simulink model "FAST_EMPC"  (R2021a)
settings: Solver=ode4  StartTime=0.0  StopTime=TMax  FixedStep=DT  MaxStep=DT  RelTol=1e-3  EnableMultiTasking=on
values from neighbouring files (symbols this model uses):
  Drivetrain =     [NREL5MW.mat]
  luenGainDisc = place(sys_tower_fa_d_obsv.A',sys_tower_fa_d_obsv.C',luenPolesDisc)'    [Init_FAST_EMPC.m]
  Parameters =     [Parameters.mat]
  RPM_Init = 9.4965    [Init_FAST_EMPC.m]
  sys_tower_fa_d_obsv = c2d(sys_tower_ss_obsv,Parameters.TsObsv,'tustin')    [Init_FAST_EMPC.m]
  sys_tower_fa_d_obsv_mode = c2d(sys_tower_ss_obsv_mode,Parameters.TsObsv,'tustin')    [Init_FAST_EMPC.m]
undefined symbols (not defined in the file or in its folder): EMPCController_Tower, luenGainDisc2, luenGainDisc_comp, OutList, strmatch, sys_tower_fa_d_obsv2, sys_tower_fa_d_obsv_comp
libraries: dspstat3 x8
(part 1 of 2)
settings Model: PauseTimes=360  Creator=bjonkman  LastModifiedBy=zfeng1
settings SolverCC: AlgebraicLoopSolver=TrustRegion
settings DataIOCC: LimitDataPoints=on  SaveFormat=Array  SignalLoggingSaveFormat=ModelDataLogs  SaveOutput=off  SaveTime=off  ReturnWorkspaceOutputs=off  SignalLoggingName=sigsOut  LoggingToFile=on  LoggingFileName=FAST_EMPC_log/220905/[220905][171055]sim_log.mat
settings OptimizationCC: ExpressionDepthLimit=2147483647  LifeSpan=inf
settings DebuggingCC: SaveWithParameterizedLinksMsg=none  UnderspecifiedInitializationDetection=Classic  MergeDetectMultiDrivingBlocksExec=none  SignalResolutionControl=TryResolveAllWithWarning  MultiTaskDSMMsg=warning  MultiTaskCondExecSysMsg=none  MultiTaskRateTransMsg=warning  FcnCallInpInsideContextMsg=warning  StateNameClashWarn=warning  SFUnexpectedBacktrackingDiag=warning  SFNoUnconditionalDefaultTransitionDiag=warning  SFExecutionAtInitializationDiag=none  SFMachineParentedDataDiag=warning  ArithmeticOperatorsInVariantConditions=warning
settings HardwareCC: ProdBitPerPointer=32  ProdBitPerSizeT=32  ProdBitPerPtrDiffT=32  ProdLargestAtomicFloat=None  ProdIntDivRoundTo=Undefined  ProdEndianess=Unspecified  ProdWordSize=32  ProdHWDeviceType=32-bit Generic  TargetUnknown=on
settings ModelReferenceCC: PropagateSignalLabelsOutOfModel=off
settings SFSimCC: SimUseLocalCustomCode=off  CustomCodeUndefinedFunction=UseInterfaceOnly
settings RTWCC: RTWUseLocalCustomCode=off
settings CodeAppCC: StateflowObjectComments=on
settings GRTTargetCC: TargetLangStandard=C89/C90 (ANSI)  CombineOutputUpdateFcns=off  GRTInterface=on
settings ConfigComp: CovMetricSettings=dw  CovSaveCumulativeToWorkspaceVar=on  CovSaveSingleToWorkspaceVar=on  CovExternalEMLEnable=off

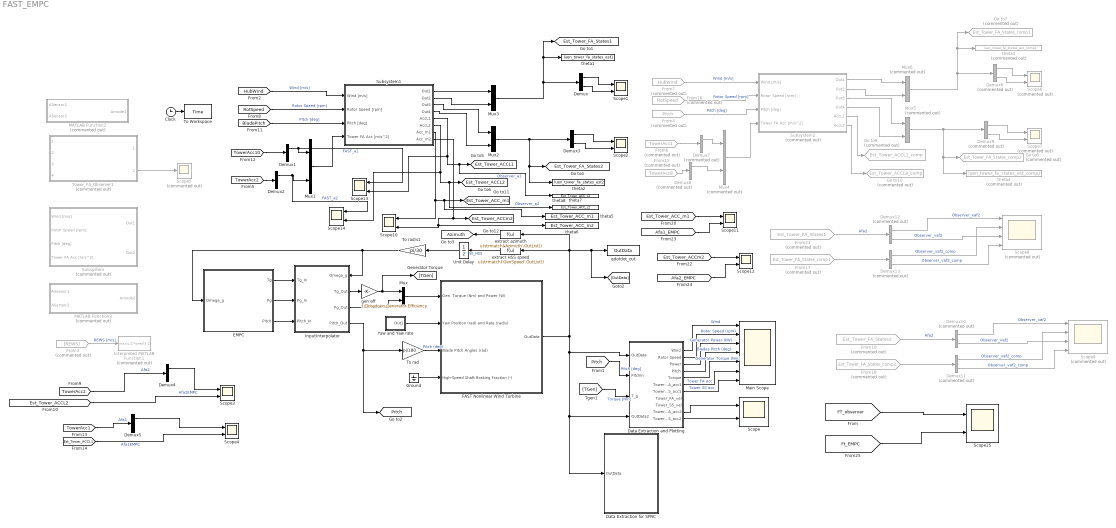
== system FAST_EMPC ==
  Clock : Clock
  Data Extraction and Plotting : Subsystem
  Data Extraction for SPRC : Subsystem
  Demux{,1..5} (6 alike) : Demux  Outputs=2
  Demux{6..13} (8 alike) : Demux  Commented=on  Outputs=2
  EMPC : Subsystem
  FAST Nonlinear Wind Turbine : Subsystem  mask(FAST Nonlinear Wind Turbine){}
      mask help: This block contains the FAST S-Function.
      mask init:
      | clear FAST_SFunc
  From15 : From  Commented=on  GotoTag=TowerAcc8  TagVisibility=global
  From16 : From  Commented=on  GotoTag=RotSpeed  TagVisibility=global
  From17 : From  Commented=on  GotoTag=Est_Tower_FA_States_comp1  TagVisibility=global
  From18 : From  Commented=on  GotoTag=Est_Tower_FA_States_comp2  TagVisibility=global
  From19 : From  Commented=on  GotoTag=Est_Tower_FA_States2  TagVisibility=global
  From21 : From  Commented=on  GotoTag=Est_Tower_FA_States1  TagVisibility=global
  From3 : From  Commented=on  GotoTag=REWS  TagVisibility=global
  From4 : From  Commented=on  GotoTag=Pitch  TagVisibility=global
  From6 : From  Commented=on  GotoTag=TowerAcc1  TagVisibility=global
  From7 : From  Commented=on  GotoTag=HubWind  TagVisibility=global
  Go to10 : Goto  Commented=on  GotoTag=Est_Tower_ACCL8_comp  TagVisibility=global
  Go to7 : Goto  Commented=on  GotoTag=Est_Tower_FA_States_comp1  TagVisibility=global
  Go to8 : Goto  Commented=on  GotoTag=Est_Tower_FA_States_comp2  TagVisibility=global
  Go to9 : Goto  Commented=on  GotoTag=Est_Tower_ACCL1_comp  TagVisibility=global
  Ground : Ground
  InputInterpolator : Subsystem
      settings: PortSchema="{\"entries\":[{\"content\":{\"sides\":[{\"content\":{\"connectorIds\":[\"In1\",\"In2\",\"In3\"]},\"type\":\"ConnectorPlacement.EquallySpacedRectSide\",\"uuid\":\"eea9236e-1f3f-4277-abdd-d5dd724ebb06\"},{\"content\":{\"connectorIds\":[\"In4\",\"Out1\",\"Out2\",\"Out3\"],\"side\":\"RIGHT\"},\"type\":\"ConnectorPlacement.EquallySpacedRectSide\",\"uuid\":\"af4b7fb0-ea5a-4e1a-9e28-eb831b9d8a57\"},{\"content\":{\"connectorIds\":[],\"side\":\"TOP\"},\"type\":\"ConnectorPlacement.EquallySpacedRectSide\",\"uuid\":\"835f85ff-c21c-4848-971b-3562e8e2ecd8\"},{\"content\":{\"connectorIds\":[],\"side\":\"BOTTOM\"},\"type\":\"ConnectorPlacement.EquallySpacedRectSide\",\"uuid\":\"cf59863e-7ec1-458a-af15-cb3c9fb145f1\"}]},\"type\":\"ConnectorPlacement.EquallySpacedConnector\",\"uuid\":\"4273e109-3171-481c-9f40-fed22461b3da\"}],\"packageUris\":[\"http://schema.mathworks.com/mf0/Connector/R2020b\"],\"version\":\"1.0\"}"
  Interpreted MATLAB Function1 : MATLABFcn  Commented=on  MATLABFcn=max(u,4)*ones(3,1)  OutputDimensions=3
  MATLAB Function2 : MATLAB Function  Commented=on  TreatAsAtomicUnit=on
  MATLAB Function3 : MATLAB Function  Commented=on  TreatAsAtomicUnit=on
  Main Scope : Scope  NumInputPorts=7
      settings: Tag=Scope
  Mux{,1..3} (4 alike) : Mux  Inputs=2
  Mux4 : Mux  Commented=on  Inputs=2
  Mux5 : Mux  Commented=on  Inputs=2
  Mux6 : Mux  Commented=on  Inputs=2
  Scope{,1..4,10..15} (11 alike) : Scope  NumInputPorts=2
  Scope5 : Scope  Commented=on
  Scope6 : Scope  Commented=on  NumInputPorts=2
  Scope7 : Scope  Commented=on  NumInputPorts=2
  Scope8 : Scope  Commented=on  NumInputPorts=4
  Scope9 : Scope  Commented=on  NumInputPorts=4
  Subsystem : Subsystem  Commented=on
  Subsystem1 : Subsystem
  Subsystem2 : Subsystem  Commented=on
  To Workspace : ToWorkspace  VariableName=Time  SampleTime=-1
  To rad : Gain  Gain=pi/180
  To rad/s1 : Gain  Gain=pi/30
  Tower_FA_Observer1 : Subsystem  Commented=on  ReferencedSubsystem=Luenberger_Tower_FA_Observer
  Unit Delay : UnitDelay  InitialCondition=RPM_Init*Drivetrain.Gearbox.Ratio  SampleTime=-1  HasFrameUpgradeWarning=on
  Yaw and Yaw rate : Subsystem
  extract HSS speed : Fcn  Expr=u(strmatch('GenSpeed',OutList))
  extract azimuth : Fcn  Expr=u(strmatch('Azimuth',OutList))
  gen eff : Gain  Gain=1/Drivetrain.Generator.Efficiency
  qdotdot_out : ToWorkspace  VariableName=OutData  SampleTime=-1
  theta1 : ToWorkspace  VariableName=luen_tower_fa_states_est1  SaveFormat=Structure With Time  SampleTime=-1
      settings: MaxDataPoints=Inf  Decimation=3
  theta2 : ToWorkspace  VariableName=luen_tower_fa_states_est2  SaveFormat=Structure With Time  SampleTime=-1
      settings: MaxDataPoints=Inf  Decimation=3
  theta3 : ToWorkspace  Commented=on  VariableName=luen_tower_fa_states_est_comp1  SaveFormat=Structure With Time  SampleTime=-1
      settings: MaxDataPoints=Inf  Decimation=3
  theta4 : ToWorkspace  Commented=on  VariableName=luen_tower_fa_states_est_comp2  SaveFormat=Structure With Time  SampleTime=-1
      settings: MaxDataPoints=Inf  Decimation=3
  theta5 : ToWorkspace  VariableName=Est_Tower_ACC_m1  SaveFormat=Structure With Time  SampleTime=-1
      settings: MaxDataPoints=Inf  Decimation=3
  theta6 : ToWorkspace  VariableName=Est_Tower_ACC_m2  SaveFormat=Structure With Time  SampleTime=-1
      settings: MaxDataPoints=Inf  Decimation=3
  theta7 : ToWorkspace  VariableName=Est_Tower_ACC_L1  SaveFormat=Structure With Time  SampleTime=-1
      settings: MaxDataPoints=Inf  Decimation=3
  theta8 : ToWorkspace  VariableName=Est_Tower_ACC_L2  SaveFormat=Structure With Time  SampleTime=-1
      settings: MaxDataPoints=Inf  Decimation=3
  tag scope: Azimuth=global, Est_Tower_ACCL1=global, Est_Tower_ACCL2=global, Est_Tower_ACC_m1=global, Est_Tower_ACCm2=global, Est_Tower_FA_States1=global, Est_Tower_FA_States2=global, Pitch=global
  wires:
  Clock/1 -> To Workspace/1
  Ground/1 -> FAST Nonlinear Wind Turbine/4(High-Speed Shaft Braking Fraction (-))
  Yaw and Yaw rate/1(Out1) -> FAST Nonlinear Wind Turbine/2(Yaw Position (rad) and Rate (rad/s))
  Mux/1 -> FAST Nonlinear Wind Turbine/1(Gen. Torque (Nm) and Power (W))
  Data Extraction and Plotting/7(Tower_SS_acc1) -> Main Scope/7  "Tower SS acc"
  Data Extraction and Plotting/2(Rotor Speed) -> Main Scope/2  "Rotor Speed (rpm)"
  Data Extraction and Plotting/3(Power) -> Main Scope/3  "Generator Power (kW)"
  Data Extraction and Plotting/4(Pitch) -> Main Scope/4  "Blades Pitch (deg)"
  Data Extraction and Plotting/5(Torque) -> Main Scope/5  "Generator Torque (Nm)"
  Data Extraction and Plotting/6(Tower_FA_acc1) -> Main Scope/6  "Tower FA acc"
  [TGen] -> Data Extraction and Plotting/3(T_g)  "Torque [Nm]"
  Data Extraction and Plotting/1(Wind) -> Main Scope/1  "Wind"
  [Pitch] -> Data Extraction and Plotting/2(PitchIn)  "Pitch [deg]"
  Unit Delay/1 -> To rad/s1/1
  extract azimuth/1 -> [Azimuth]
  extract HSS speed/1 -> Unit Delay/1  "W_HSS"
  To rad/s1/1 -> EMPC/1(Omega_g), InputInterpolator/4(Omega_g)
  InputInterpolator/1(Tg_Out) -> gen eff/1
  gen eff/1 -> Mux/1, [TGen]
  InputInterpolator/2(Pg_Out) -> Mux/2
  To rad/1 -> FAST Nonlinear Wind Turbine/3(Blade Pitch Angles (rad))  "Pitch (deg)"
  InputInterpolator/3(Pitch_Out) -> [Pitch], To rad/1
  EMPC/1(Tg) -> InputInterpolator/1(Tg_In)
  EMPC/2(Pg) -> InputInterpolator/2(Pg_In)
  EMPC/3(Pitch) -> InputInterpolator/3(Pitch_In)
  [RotSpeed] -> Subsystem1/2(Rotor Speed [rpm])  "Rotor Speed [rpm]"
  [HubWind] -> Subsystem1/1(Wind [m/s])  "Wind [m/s]"
  Subsystem1/1(Out1) -> Mux3/1
  Subsystem1/2(Out2) -> Mux3/2
  Mux3/1 -> Demux/1, [Est_Tower_FA_States1], theta1/1
  From3/1 -> Interpreted MATLAB Function1/1  "REWS [m/s]"
  FAST Nonlinear Wind Turbine/1(OutData) -> Data Extraction for SPRC/1(OutData), Data Extraction and Plotting/4(OutData2), Data Extraction and Plotting/1(OutData), extract azimuth/1, extract HSS speed/1, [OutData], qdotdot_out/1
  Data Extraction and Plotting/10(Tower_FA_acc2) -> Scope/1
  Data Extraction and Plotting/11(Tower_SS_acc2) -> Scope/2
  Demux3/1 -> Scope2/1
  Demux3/2 -> Scope2/2
  Demux/1 -> Scope1/1
  Demux/2 -> Scope1/2
  [TowerAcc2] -> Demux4/1  "Afa2"
  [Est_Tower_ACCL2] -> Scope3/2  "Afa2EMPC"
  [TowerAcc1] -> Demux5/1  "Afa1"
  [Est_Tower_ACCL1] -> Scope4/2  "Afa1EMPC"
  Tower_FA_Observer1/2 -> Scope5/1
  [BladePitch] -> Subsystem1/3(Pitch [deg])  "Pitch [deg]"
  Mux1/1 -> Subsystem1/4(Tower FA Acc [m/s^2])
  [TowerAcc10] -> Demux1/1
  [TowerAcc2] -> Demux2/1
  Subsystem1/4(Out4) -> Mux2/2
  Subsystem1/3(Out3) -> Mux2/1
  Mux2/1 -> theta2/1, [Est_Tower_FA_States2], Demux3/1
  Demux2/1 -> Scope14/1, Mux1/2  "FAST_a2"
  Demux1/1 -> Scope13/1, Mux1/1  "FAST_a1"
  Subsystem1/5(AccL1) -> Scope13/2, theta7/1, [Est_Tower_ACCL1]  "Observer_a1"
  Subsystem1/6(AccL2) -> Scope14/2, theta8/1, [Est_Tower_ACCL2]  "Observer_a2"
  Demux4/1 -> Scope3/1
  Demux5/1 -> Scope4/1
  Subsystem2/6(AccL2) -> Go to10/1
  Subsystem2/5(AccL1) -> Go to9/1
  Demux8/1 -> Mux4/2
  From6/1 -> Demux7/1
  Subsystem2/4(Out4) -> Mux5/2
  From15/1 -> Demux8/1
  Subsystem2/3(Out3) -> Mux5/1
  Mux4/1 -> Subsystem2/4(Tower FA Acc [m/s^2])
  Mux5/1 -> theta4/1, Go to8/1, Demux9/1
  Subsystem2/2(Out2) -> Mux6/2
  Subsystem2/1(Out1) -> Mux6/1
  Demux7/1 -> Mux4/1
  From4/1 -> Subsystem2/3(Pitch [deg])  "Pitch [deg]"
  From16/1 -> Subsystem2/2(Rotor Speed [rpm])  "Rotor Speed [rpm]"
  From7/1 -> Subsystem2/1(Wind [m/s])  "Wind [m/s]"
  Demux9/1 -> Scope7/1
  Demux6/1 -> Scope6/1
  Mux6/1 -> Demux6/1, Go to7/1, theta3/1
  Demux6/2 -> Scope6/2
  Demux9/2 -> Scope7/2
  From17/1 -> Demux13/1
  From21/1 -> Demux12/1  "Afa2"
  Demux12/1 -> Scope8/1  "Observer_xaf2"
  Demux13/1 -> Scope8/2  "Observer_xaf2_comp"
  Demux12/2 -> Scope8/3  "Observer_vaf2"
  Demux13/2 -> Scope8/4  "Observer_vaf2_comp"
  Demux11/2 -> Scope9/4  "Observer_vaf2_comp"
  Demux10/1 -> Scope9/1  "Observer_xaf2"
  From19/1 -> Demux10/1  "Afa2"
  Demux11/1 -> Scope9/2  "Observer_xaf2_comp"
  From18/1 -> Demux11/1
  Demux10/2 -> Scope9/3  "Observer_vaf2"
  Subsystem1/7(Acc_m1) -> theta5/1, [Est_Tower_ACC_m1], Scope10/1
  [Est_Tower_ACC_m1] -> Scope11/1
  [Est_Tower_ACCm2] -> Scope12/1
  [Afa1_EMPC] -> Scope11/2
  [Afa2_EMPC] -> Scope12/2
  Subsystem1/8(Acc_m2) -> [Est_Tower_ACCm2], Scope10/2, theta6/1
  [FT_observer] -> Scope15/1
  [Ft_EMPC] -> Scope15/2

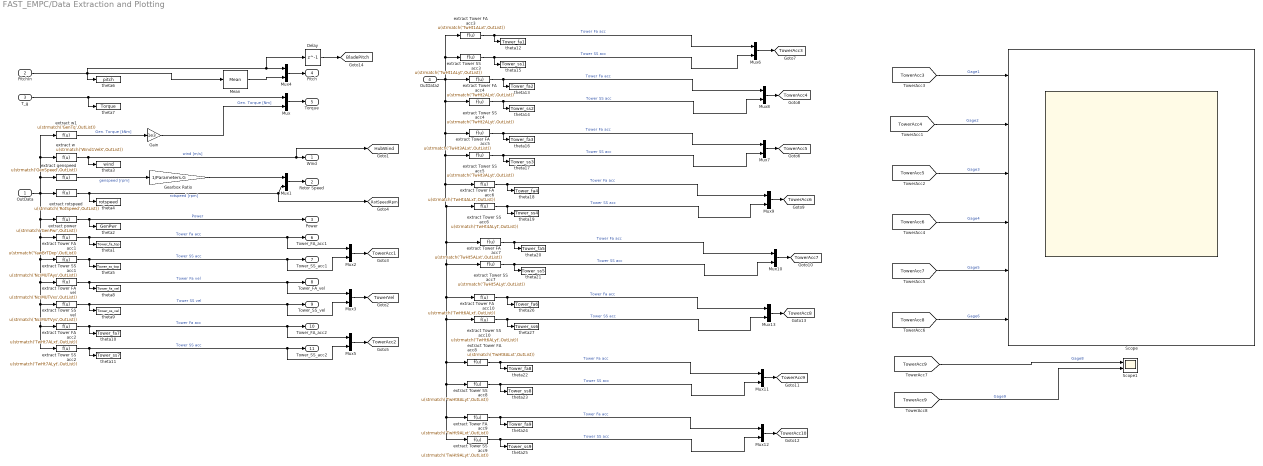
== system FAST_EMPC/Data Extraction and Plotting ==
  OutData : Inport
  PitchIn : Inport  Port=2
  T_g : Inport  Port=3
  OutData2 : Inport  Port=4
  Delay : Delay  DelayLength=1  InitialCondition=0
  Gain : Gain  Gain=1e3
  Gearbox Ratio : Gain  Gain=1/Parameters.G
  Mean : dspstat3/Mean  run=off  InputProcessing=Columns as channels (frame based)  reset_popup=None  directionMode=Each column  dimension=1  roiEnable=off  roiType=Rectangles  roiPortion=Entire ROI  roiOutput=Individual statistics for each ROI  roiFlag=off  roundingMode=Floor  overflowMode=off  outputDataTypeStr=Inherit: Same as accumulator  outputMin=[]  outputMax=[]  outputLastDataTypeStr=Inherit: Same as accumulator
  Mux{,1..13} (14 alike) : Mux  Inputs=2
  Scope : Scope  NumInputPorts=6
  Scope1 : Scope  NumInputPorts=2
  extract Tower FA acc1 : Fcn  Expr=u(strmatch('YawBrTDxp',OutList))
  extract Tower FA acc10 : Fcn  Expr=u(strmatch('TwHt6ALxt',OutList))
  extract Tower FA acc2 : Fcn  Expr=u(strmatch('TwHt7ALxt',OutList))
  extract Tower FA acc3 : Fcn  Expr=u(strmatch('TwHt1ALxt',OutList))
  extract Tower FA acc4 : Fcn  Expr=u(strmatch('TwHt2ALxt',OutList))
  extract Tower FA acc5 : Fcn  Expr=u(strmatch('TwHt3ALxt',OutList))
  extract Tower FA acc6 : Fcn  Expr=u(strmatch('TwHt4ALxt',OutList))
  extract Tower FA acc7 : Fcn  Expr=u(strmatch('TwHt5ALxt',OutList))
  extract Tower FA acc8 : Fcn  Expr=u(strmatch('TwHt8ALxt',OutList))
  extract Tower FA acc9 : Fcn  Expr=u(strmatch('TwHt9ALxt',OutList))
  extract Tower FA vel : Fcn  Expr=u(strmatch('NcIMUTVxs',OutList))
  extract Tower SS acc1 : Fcn  Expr=u(strmatch('NcIMUTAys',OutList))
  extract Tower SS acc10 : Fcn  Expr=u(strmatch('TwHt6ALyt',OutList))
  extract Tower SS acc2 : Fcn  Expr=u(strmatch('TwHt7ALyt',OutList))
  extract Tower SS acc3 : Fcn  Expr=u(strmatch('TwHt1ALyt',OutList))
  extract Tower SS acc4 : Fcn  Expr=u(strmatch('TwHt2ALyt',OutList))
  extract Tower SS acc5 : Fcn  Expr=u(strmatch('TwHt3ALyt',OutList))
  extract Tower SS acc6 : Fcn  Expr=u(strmatch('TwHt4ALyt',OutList))
  extract Tower SS acc7 : Fcn  Expr=u(strmatch('TwHt5ALyt',OutList))
  extract Tower SS acc8 : Fcn  Expr=u(strmatch('TwHt8ALyt',OutList))
  extract Tower SS acc9 : Fcn  Expr=u(strmatch('TwHt9ALyt',OutList))
  extract Tower SS vel : Fcn  Expr=u(strmatch('NcIMUTVys',OutList))
  extract genspeed : Fcn  Expr=u(strmatch('GenSpeed',OutList))
  extract power : Fcn  Expr=u(strmatch('GenPwr',OutList))
  extract rotspeed : Fcn  Expr=u(strmatch('RotSpeed',OutList))
  extract w : Fcn  Expr=u(strmatch('Wind1VelX',OutList))
  extract w1 : Fcn  Expr=u(strmatch('GenTq',OutList))
  theta1 : ToWorkspace  VariableName=Tower_fa_top  SaveFormat=Structure With Time  SampleTime=-1
      settings: MaxDataPoints=Inf  Decimation=3
  theta10 : ToWorkspace  VariableName=Tower_fa7  SaveFormat=Structure With Time  SampleTime=-1
      settings: MaxDataPoints=Inf  Decimation=3
  theta11 : ToWorkspace  VariableName=Tower_ss7  SaveFormat=Structure With Time  SampleTime=-1
      settings: MaxDataPoints=Inf  Decimation=3
  theta12 : ToWorkspace  VariableName=Tower_fa1  SaveFormat=Structure With Time  SampleTime=-1
      settings: MaxDataPoints=Inf  Decimation=3
  theta13 : ToWorkspace  VariableName=Tower_fa2  SaveFormat=Structure With Time  SampleTime=-1
      settings: MaxDataPoints=Inf  Decimation=3
  theta14 : ToWorkspace  VariableName=Tower_ss2  SaveFormat=Structure With Time  SampleTime=-1
      settings: MaxDataPoints=Inf  Decimation=3
  theta15 : ToWorkspace  VariableName=Tower_ss1  SaveFormat=Structure With Time  SampleTime=-1
      settings: MaxDataPoints=Inf  Decimation=3
  theta16 : ToWorkspace  VariableName=Tower_fa3  SaveFormat=Structure With Time  SampleTime=-1
      settings: MaxDataPoints=Inf  Decimation=3
  theta17 : ToWorkspace  VariableName=Tower_ss3  SaveFormat=Structure With Time  SampleTime=-1
      settings: MaxDataPoints=Inf  Decimation=3
  theta18 : ToWorkspace  VariableName=Tower_fa4  SaveFormat=Structure With Time  SampleTime=-1
      settings: MaxDataPoints=Inf  Decimation=3
  theta19 : ToWorkspace  VariableName=Tower_ss4  SaveFormat=Structure With Time  SampleTime=-1
      settings: MaxDataPoints=Inf  Decimation=3
  theta2 : ToWorkspace  VariableName=GenPwr  SaveFormat=Structure With Time  SampleTime=-1
      settings: MaxDataPoints=Inf  Decimation=3
  theta20 : ToWorkspace  VariableName=Tower_fa5  SaveFormat=Structure With Time  SampleTime=-1
      settings: MaxDataPoints=Inf  Decimation=3
  theta21 : ToWorkspace  VariableName=Tower_ss5  SaveFormat=Structure With Time  SampleTime=-1
      settings: MaxDataPoints=Inf  Decimation=3
  theta22 : ToWorkspace  VariableName=Tower_fa8  SaveFormat=Structure With Time  SampleTime=-1
      settings: MaxDataPoints=Inf  Decimation=3
  theta23 : ToWorkspace  VariableName=Tower_ss8  SaveFormat=Structure With Time  SampleTime=-1
      settings: MaxDataPoints=Inf  Decimation=3
  theta24 : ToWorkspace  VariableName=Tower_fa9  SaveFormat=Structure With Time  SampleTime=-1
      settings: MaxDataPoints=Inf  Decimation=3
  theta25 : ToWorkspace  VariableName=Tower_ss9  SaveFormat=Structure With Time  SampleTime=-1
      settings: MaxDataPoints=Inf  Decimation=3
  theta26 : ToWorkspace  VariableName=Tower_fa6  SaveFormat=Structure With Time  SampleTime=-1
      settings: MaxDataPoints=Inf  Decimation=3
  theta27 : ToWorkspace  VariableName=Tower_ss6  SaveFormat=Structure With Time  SampleTime=-1
      settings: MaxDataPoints=Inf  Decimation=3
  theta3 : ToWorkspace  VariableName=wind  SaveFormat=Structure With Time  SampleTime=-1
      settings: MaxDataPoints=Inf  Decimation=3
  theta4 : ToWorkspace  VariableName=rotspeed  SaveFormat=Structure With Time  SampleTime=-1
      settings: MaxDataPoints=Inf  Decimation=3
  theta5 : ToWorkspace  VariableName=Tower_ss_top  SaveFormat=Structure With Time  SampleTime=-1
      settings: MaxDataPoints=Inf  Decimation=3
  theta6 : ToWorkspace  VariableName=pitch  SaveFormat=Structure With Time  SampleTime=-1
      settings: MaxDataPoints=Inf  Decimation=3
  theta7 : ToWorkspace  VariableName=Torque  SaveFormat=Structure With Time  SampleTime=-1
      settings: MaxDataPoints=Inf  Decimation=3
  theta8 : ToWorkspace  VariableName=Tower_fa_vel  SaveFormat=Structure With Time  SampleTime=-1
      settings: MaxDataPoints=Inf  Decimation=3
  theta9 : ToWorkspace  VariableName=Tower_ss_vel  SaveFormat=Structure With Time  SampleTime=-1
      settings: MaxDataPoints=Inf  Decimation=3
  Wind : Outport  VectorParamsAs1DForOutWhenUnconnected=off
  Rotor Speed : Outport  Port=2  VectorParamsAs1DForOutWhenUnconnected=off
  Power : Outport  Port=3  VectorParamsAs1DForOutWhenUnconnected=off
  Pitch : Outport  Port=4  VectorParamsAs1DForOutWhenUnconnected=off
  Torque : Outport  Port=5  VectorParamsAs1DForOutWhenUnconnected=off
  Tower_FA_acc1 : Outport  Port=6  VectorParamsAs1DForOutWhenUnconnected=off
  Tower_SS_acc1 : Outport  Port=7  VectorParamsAs1DForOutWhenUnconnected=off
  Tower_FA_vel : Outport  Port=8  VectorParamsAs1DForOutWhenUnconnected=off
  Tower_SS_vel : Outport  Port=9  VectorParamsAs1DForOutWhenUnconnected=off
  Tower_FA_acc2 : Outport  Port=10  VectorParamsAs1DForOutWhenUnconnected=off
  Tower_SS_acc2 : Outport  Port=11  VectorParamsAs1DForOutWhenUnconnected=off
  tag scope: BladePitch=global, HubWind=global, RotSpeedRpm=global, TowerAcc10=global, TowerAcc1=global, TowerAcc2=global, TowerAcc3=global, TowerAcc4=global, TowerAcc5=global, TowerAcc6=global, TowerAcc7=global, TowerAcc8=global, TowerAcc9=global, TowerVel=global
  wires:
  extract w/1 -> [HubWind], Wind/1, theta3/1  "wind [m/s]"
  extract rotspeed/1 -> [RotSpeedRpm], Mux1/2, theta4/1  "rotspeed [rpm]"
  extract power/1 -> theta2/1, Power/1  "Power"
  PitchIn/1 -> theta6/1, Delay/1, Mux4/1, Mean/1
  T_g/1 -> Mux/1, theta7/1
  extract Tower FA acc1/1 -> theta1/1, Tower_FA_acc1/1, Mux2/1  "Tower Fa acc"
  extract Tower SS acc1/1 -> theta5/1, Mux2/2, Tower_SS_acc1/1  "Tower SS acc"
  extract w1/1 -> Gain/1  "Gen. Torque [kNm]"
  Gain/1 -> Mux/2  "Gen. Torque [Nm]"
  Mux/1 -> Torque/1
  Mux1/1 -> Rotor Speed/1
  extract genspeed/1 -> Gearbox Ratio/1  "genspeed [rpm]"
  Gearbox Ratio/1 -> Mux1/1
  extract Tower SS vel/1 -> Mux3/2, Tower_SS_vel/1, theta9/1  "Tower SS vel"
  extract Tower FA vel/1 -> Mux3/1, Tower_FA_vel/1, theta8/1  "Tower Fa vel"
  Mux2/1 -> [TowerAcc1]
  Mux3/1 -> [TowerVel]
  Mux4/1 -> Pitch/1
  Mean/1 -> Mux4/2
  OutData/1 -> extract Tower FA vel/1, extract Tower SS acc2/1, extract Tower FA acc2/1, extract Tower SS vel/1, extract Tower SS acc1/1, extract Tower FA acc1/1, extract power/1, extract w1/1, extract w/1, extract genspeed/1, extract rotspeed/1
  extract Tower SS acc2/1 -> theta11/1, Mux5/2, Tower_SS_acc2/1  "Tower SS acc"
  extract Tower FA acc2/1 -> theta10/1, Tower_FA_acc2/1, Mux5/1  "Tower Fa acc"
  Mux5/1 -> [TowerAcc2]
  Mux8/1 -> [TowerAcc4]
  extract Tower FA acc4/1 -> theta13/1, Mux8/1  "Tower Fa acc"
  extract Tower SS acc3/1 -> theta15/1, Mux6/2  "Tower SS acc"
  extract Tower FA acc3/1 -> theta12/1, Mux6/1  "Tower Fa acc"
  Mux6/1 -> [TowerAcc3]
  extract Tower SS acc4/1 -> theta14/1, Mux8/2  "Tower SS acc"
  extract Tower SS acc5/1 -> theta17/1, Mux7/2  "Tower SS acc"
  Mux7/1 -> [TowerAcc5]
  extract Tower FA acc5/1 -> theta16/1, Mux7/1  "Tower Fa acc"
  extract Tower FA acc6/1 -> theta18/1, Mux9/1  "Tower Fa acc"
  Mux9/1 -> [TowerAcc6]
  extract Tower SS acc6/1 -> theta19/1, Mux9/2  "Tower SS acc"
  extract Tower SS acc7/1 -> theta21/1, Mux10/2  "Tower SS acc"
  Mux10/1 -> [TowerAcc7]
  extract Tower FA acc7/1 -> theta20/1, Mux10/1  "Tower Fa acc"
  extract Tower SS acc8/1 -> theta23/1, Mux11/2  "Tower SS acc"
  extract Tower FA acc8/1 -> theta22/1, Mux11/1  "Tower Fa acc"
  Mux11/1 -> [TowerAcc9]
  Mux12/1 -> [TowerAcc10]
  extract Tower SS acc9/1 -> theta25/1, Mux12/2  "Tower SS acc"
  extract Tower FA acc9/1 -> theta24/1, Mux12/1  "Tower Fa acc"
  [TowerAcc3] -> Scope/1  "Gage1"
  [TowerAcc4] -> Scope/2  "Gage2"
  [TowerAcc5] -> Scope/3  "Gage3"
  [TowerAcc6] -> Scope/4  "Gage4"
  [TowerAcc7] -> Scope/5  "Gage5"
  [TowerAcc8] -> Scope/6  "Gage6"
  [TowerAcc9] -> Scope1/1  "Gage8"
  extract Tower SS acc10/1 -> theta27/1, Mux13/2  "Tower SS acc"
  extract Tower FA acc10/1 -> theta26/1, Mux13/1  "Tower Fa acc"
  OutData2/1 -> extract Tower FA acc4/1, extract Tower FA acc6/1, extract Tower SS acc9/1, extract Tower FA acc9/1, extract Tower SS acc8/1, extract Tower FA acc8/1, extract Tower SS acc10/1, extract Tower FA acc10/1, extract Tower SS acc7/1, extract Tower FA acc7/1, extract Tower SS acc6/1, extract Tower SS acc5/1, extract Tower FA acc5/1, extract Tower SS acc4/1, extract Tower FA acc3/1, extract Tower SS acc3/1
  Mux13/1 -> [TowerAcc8]
  [TowerAcc9] -> Scope1/2  "Gage9"
  Delay/1 -> [BladePitch]

== system FAST_EMPC/Data Extraction for SPRC ==
  OutData : Inport
  extract RtVAvgxh : Fcn  Expr=u(strmatch('RtVAvgxh',OutList))
  extract rotPower : Fcn  Expr=u(strmatch('RotPwr',OutList))
  extract rotspeed : Fcn  Expr=u(strmatch('RotSpeed',OutList))
  tag scope: RotPower=global, RotSpeed=global, RtVAvgxh=global
  wires:
  extract rotPower/1 -> [RotPower]  "rotPower [kW]"
  OutData/1 -> extract rotPower/1, extract RtVAvgxh/1, extract rotspeed/1
  extract RtVAvgxh/1 -> [RtVAvgxh]  "wind [m/s]"
  extract rotspeed/1 -> [RotSpeed]  "rotspeed [rpm]"

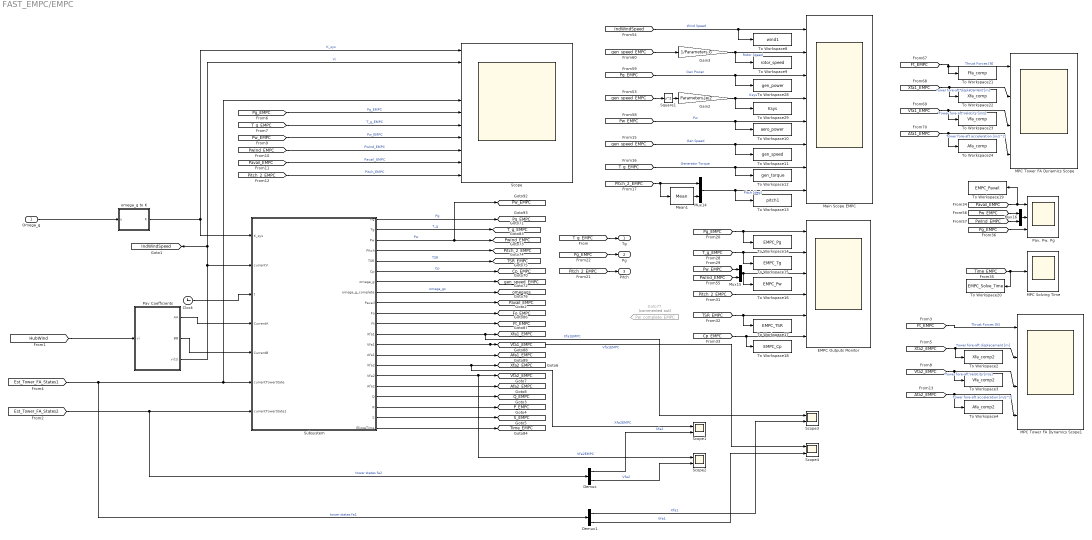
== system FAST_EMPC/EMPC ==
  Omega_g : Inport
  Clock : Clock
  Demux : Demux  Outputs=2
  Demux1 : Demux  Outputs=2
  EMPC Outputs Monitor : Scope  NumInputPorts=6
  Gain2 : Gain  Gain=Parameters.Je/2
  Gain3 : Gain  Gain=1/Parameters.G
  Goto77 : Goto  Commented=on  GotoTag=Pw_complete_EMPC  TagVisibility=global
  MPC Solving Time : Scope
  MPC Tower FA Dynamics Scope : Scope  NumInputPorts=4
  MPC Tower FA Dynamics Scope1 : Scope  NumInputPorts=4
  Main Scope EMPC : Scope  NumInputPorts=8
  Mean1 : dspstat3/Mean  run=off  InputProcessing=Columns as channels (frame based)  reset_popup=None  directionMode=Each column  dimension=1  roiEnable=off  roiType=Rectangles  roiPortion=Entire ROI  roiOutput=Individual statistics for each ROI  roiFlag=off  roundingMode=Floor  overflowMode=off  outputDataTypeStr=Inherit: Same as accumulator  outputMin=[]  outputMax=[]  outputLastDataTypeStr=Inherit: Same as accumulator
  Mux14 : Mux  Inputs=2
  Mux15 : Mux  Inputs=2
  Mux16 : Mux  Inputs=2
  Pav Coefficients : Subsystem
  "Pav, Pw, Pg" : Scope  NumInputPorts=3
  Scope : Scope  NumInputPorts=11
  Scope{1..4} (4 alike) : Scope  NumInputPorts=2
  Square1 : Math  Operator=square  SaturateOnIntegerOverflow=on
  Subsystem : Subsystem
  To Workspace10 : ToWorkspace  VariableName=aero_power  SaveFormat=Structure With Time  SampleTime=-1
  To Workspace11 : ToWorkspace  VariableName=gen_speed  SaveFormat=Structure With Time  SampleTime=-1
  To Workspace12 : ToWorkspace  VariableName=gen_torque  SaveFormat=Structure With Time  SampleTime=-1
  To Workspace13 : ToWorkspace  VariableName=pitch1  SaveFormat=Structure With Time  SampleTime=-1
  To Workspace14 : ToWorkspace  VariableName=EMPC_Pg  SaveFormat=Structure With Time  SampleTime=-1
  To Workspace15 : ToWorkspace  VariableName=EMPC_Tg  SaveFormat=Structure With Time  SampleTime=-1
  To Workspace16 : ToWorkspace  VariableName=EMPC_Pw  SaveFormat=Structure With Time  SampleTime=-1
  To Workspace17 : ToWorkspace  VariableName=EMPC_TSR  SaveFormat=Structure With Time  SampleTime=-1
  To Workspace18 : ToWorkspace  VariableName=EMPC_Cp  SaveFormat=Structure With Time  SampleTime=-1
  To Workspace19 : ToWorkspace  VariableName=EMPC_Pavail  SaveFormat=Structure With Time  SampleTime=-1
  To Workspace2 : ToWorkspace  VariableName=Xfa_comp2  SaveFormat=Structure With Time  SampleTime=-1
  To Workspace20 : ToWorkspace  VariableName=EMPC_Solve_Time  SaveFormat=Structure With Time  SampleTime=-1
  To Workspace21 : ToWorkspace  VariableName=Ffa_comp  SaveFormat=Structure With Time  SampleTime=-1
  To Workspace22 : ToWorkspace  VariableName=Xfa_comp  SaveFormat=Structure With Time  SampleTime=-1
  To Workspace23 : ToWorkspace  VariableName=Vfa_comp  SaveFormat=Structure With Time  SampleTime=-1
  To Workspace24 : ToWorkspace  VariableName=Afa_comp  SaveFormat=Structure With Time  SampleTime=-1
  To Workspace28 : ToWorkspace  VariableName=gen_power  SaveFormat=Structure With Time  SampleTime=-1
  To Workspace29 : ToWorkspace  VariableName=Ksys  SaveFormat=Structure With Time  SampleTime=-1
  To Workspace3 : ToWorkspace  VariableName=Vfa_comp2  SaveFormat=Structure With Time  SampleTime=-1
  To Workspace4 : ToWorkspace  VariableName=Afa_comp2  SaveFormat=Structure With Time  SampleTime=-1
  To Workspace8 : ToWorkspace  VariableName=wind1  SaveFormat=Structure With Time  SampleTime=-1
  To Workspace9 : ToWorkspace  VariableName=rotor_speed  SaveFormat=Structure With Time  SampleTime=-1
  omega_g to K : MATLAB Function  TreatAsAtomicUnit=on  SystemSampleTime=Parameters.TsFAST
  Tg : Outport
  Pg : Outport  Port=2
  Pitch : Outport  Port=3
  tag scope: Afa1_EMPC=global, Afa2_EMPC=global, Cp_EMPC=global, Fo_EMPC=global, Ft_EMPC=global, IndWindSpeed=global, P_EMPC=global, Pavail_EMPC=global, Pg_EMPC=global, Pitch_2_EMPC=global, PwInd_EMPC=global, Pw_EMPC=global, Q_EMPC=global, S_EMPC=global, TSR_EMPC=global, T_g_EMPC=global, Time_EMPC=global, Vfa1_EMPC=global, Vfa2_EMPC=global, Xfa1_EMPC=global, Xfa2_EMPC=global, gen_speed_EMPC=global, omegags=global
  wires:
  omega_g to K/1(K) -> Scope/1, Subsystem/1(K_sys)  "K_sys"
  [Est_Tower_FA_States1] -> Demux1/1, Scope/5, Subsystem/6(currentTowerState)  "tower states fa1"
  Clock/1 -> Subsystem/3(t)
  Pav Coefficients/3(vi(1)) -> Scope/2, [IndWindSpeed], Subsystem/2(currentV)  "Vi"
  Pav Coefficients/2(BB) -> Subsystem/5(CurrentB)
  Pav Coefficients/1(AA) -> Subsystem/4(CurrentA)
  [Pg_EMPC] -> Scope/6  "Pg_EMPC"
  [T_g_EMPC] -> Scope/7  "T_g_EMPC"
  [Pw_EMPC] -> Scope/8  "Pw_EMPC"
  [PwInd_EMPC] -> Scope/9  "PwInd_EMPC"
  [Pavail_EMPC] -> Scope/10  "Pavail_EMPC"
  [Pitch_2_EMPC] -> Scope/11  "Pitch_EMPC"
  [Pw_EMPC] -> Mux16/1
  [Cp_EMPC] -> EMPC Outputs Monitor/6, To Workspace18/1
  Gain2/1 -> Main Scope EMPC/4, To Workspace29/1  "Ksys"
  [Pitch_2_EMPC] -> Mux14/1, Mean1/1
  [Xfa1_EMPC] -> MPC Tower FA Dynamics Scope/2, To Workspace22/1  "Tower fore-aft displacement [m]"
  [Vfa1_EMPC] -> MPC Tower FA Dynamics Scope/3, To Workspace23/1  "Tower fore-aft velocity [m/s]"
  [TSR_EMPC] -> EMPC Outputs Monitor/5, To Workspace17/1
  Square1/1 -> Gain2/1
  [PwInd_EMPC] -> Mux15/2
  Mux16/1 -> "Pav, Pw, Pg"/2
  [Pg_EMPC] -> "Pav, Pw, Pg"/3
  [Time_EMPC] -> To Workspace20/1, MPC Solving Time/1
  [Ft_EMPC] -> MPC Tower FA Dynamics Scope/1, To Workspace21/1  "Thrust Forces [N]"
  Mux14/1 -> To Workspace13/1, Main Scope EMPC/8  "Pitch [deg]"
  [Pavail_EMPC] -> To Workspace19/1, "Pav, Pw, Pg"/1
  [Pg_EMPC] -> EMPC Outputs Monitor/1, To Workspace14/1
  Mux15/1 -> EMPC Outputs Monitor/3, To Workspace16/1
  [gen_speed_EMPC] -> Gain3/1
  [Afa1_EMPC] -> MPC Tower FA Dynamics Scope/4, To Workspace24/1  "Tower fore-aft acceleration [m/s^2]"
  [Pitch_2_EMPC] -> EMPC Outputs Monitor/4
  [gen_speed_EMPC] -> To Workspace11/1, Main Scope EMPC/6  "Gen Speed"
  [IndWindSpeed] -> To Workspace8/1, Main Scope EMPC/1  "Wind Speed"
  [T_g_EMPC] -> EMPC Outputs Monitor/2, To Workspace15/1
  [Pw_EMPC] -> Main Scope EMPC/5, To Workspace10/1  "Pw"
  [T_g_EMPC] -> To Workspace12/1, Main Scope EMPC/7  "Generator Torque"
  [PwInd_EMPC] -> Mux16/2
  [gen_speed_EMPC] -> Square1/1
  [Pg_EMPC] -> Main Scope EMPC/3, To Workspace28/1  "Gen Power"
  Mean1/1 -> Mux14/2
  [Pw_EMPC] -> Mux15/1
  Gain3/1 -> Main Scope EMPC/2, To Workspace9/1  "Rotor Speed"
  [Pitch_2_EMPC] -> Pitch/1
  [Pg_EMPC] -> Pg/1
  [T_g_EMPC] -> Tg/1
  Omega_g/1 -> omega_g to K/1(u)
  [HubWind] -> Pav Coefficients/1(vi)
  Subsystem/4(Pitch) -> [Pitch_2_EMPC]
  Subsystem/19(R) -> [P_EMPC]
  Subsystem/1(Pg) -> [Pg_EMPC]  "Pg"
  Subsystem/17(Afa2) -> [Afa2_EMPC]
  Subsystem/21(ElipseTime) -> [Time_EMPC]
  Subsystem/20(S) -> [S_EMPC]
  Subsystem/10(Fo) -> [Fo_EMPC]
  Subsystem/18(Q) -> [Q_EMPC]
  Subsystem/12(Xfa1) -> Scope3/1, [Xfa1_EMPC]  "Xfa1EMPC"
  Subsystem/5(TSR) -> [TSR_EMPC]  "TSR"
  Subsystem/8(omega_g_complete) -> [omegags]  "omega_gs"
  Subsystem/9(Pavail) -> [Pavail_EMPC]
  Subsystem/11(Ft) -> [Ft_EMPC]
  Subsystem/2(Tg) -> [T_g_EMPC]  "T_g"
  Subsystem/14(Afa1) -> [Afa1_EMPC]
  Subsystem/3(Pw) -> [Pw_EMPC], [PwInd_EMPC]  "Pw"
  Subsystem/15(Xfa2) -> Scope1/1, [Xfa2_EMPC]  "Xfa2EMPC"
  Subsystem/13(Vfa1) -> Scope4/1, [Vfa1_EMPC]  "Vfa1EMPC"
  Subsystem/16(Vfa2) -> Scope2/1, [Vfa2_EMPC]  "Vfa2EMPC"
  Subsystem/6(Cp) -> [Cp_EMPC]  "Cp"
  Subsystem/7(omega_g) -> [gen_speed_EMPC]
  [Est_Tower_FA_States2] -> Demux/1, Subsystem/7(currentTowerState1)  "tower states fa2"
  [Afa2_EMPC] -> MPC Tower FA Dynamics Scope1/4, To Workspace4/1  "Tower fore-aft acceleration [m/s^2]"
  [Ft_EMPC] -> MPC Tower FA Dynamics Scope1/1  "Thrust Forces [N]"
  [Vfa2_EMPC] -> MPC Tower FA Dynamics Scope1/3, To Workspace3/1  "Tower fore-aft velocity [m/s]"
  [Xfa2_EMPC] -> MPC Tower FA Dynamics Scope1/2, To Workspace2/1  "Tower fore-aft displacement [m]"
  Demux/1 -> Scope1/2  "Xfa2"
  Demux/2 -> Scope2/2  "Vfa2"
  Demux1/1 -> Scope3/2  "Xfa1"
  Demux1/2 -> Scope4/2  "Vfa1"

== system FAST_EMPC/FAST Nonlinear Wind Turbine ==
  Gen. Torque (Nm) and Power (W) : Inport
  Yaw Position (rad) and Rate (rad/s) : Inport  Port=2
  Blade Pitch Angles (rad) : Inport  Port=3
  High-Speed Shaft Braking Fraction (-) : Inport  Port=4
  Mux1 : Mux
  S-Function : S-Function  FunctionName=FAST_SFunc  Parameters=FAST, TMax, 0  SFunctionDeploymentMode=off  EnableBusSupport=off
  Signal Specification1 : SignalSpecification  OutDataTypeStr=double  Dimensions=2
  Signal Specification2 : SignalSpecification  OutDataTypeStr=double  Dimensions=2
  OutData : Outport
  wires:
  Gen. Torque (Nm) and Power (W)/1 -> Signal Specification1/1
  S-Function/1 -> OutData/1
  Mux1/1 -> S-Function/1
  Blade Pitch Angles (rad)/1 -> Mux1/3
  Yaw Position (rad) and Rate (rad/s)/1 -> Signal Specification2/1
  Signal Specification1/1 -> Mux1/1
  Signal Specification2/1 -> Mux1/2
  High-Speed Shaft Braking Fraction (-)/1 -> Mux1/4

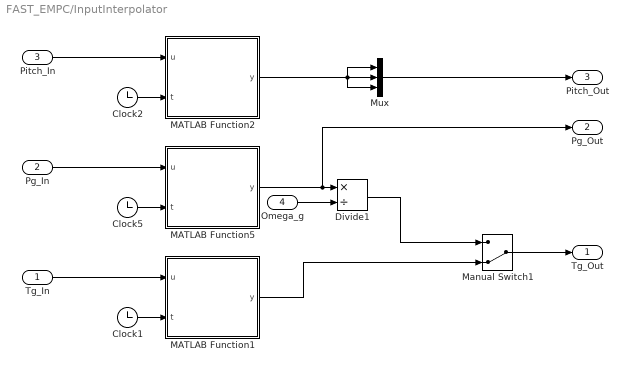
== system FAST_EMPC/InputInterpolator ==
  Tg_In : Inport
  Pg_In : Inport  Port=2
  Pitch_In : Inport  Port=3
  Omega_g : Inport  Port=4
  Clock1 : Clock
  Clock2 : Clock
  Clock5 : Clock
  Divide1 : Product  Inputs=*/
  MATLAB Function1 : MATLAB Function  TreatAsAtomicUnit=on
  MATLAB Function2 : MATLAB Function  TreatAsAtomicUnit=on
  MATLAB Function5 : MATLAB Function  TreatAsAtomicUnit=on
  Manual Switch1 : ManualSwitch  CurrentSetting=0
  Mux : Mux  Inputs=3
  Tg_Out : Outport
  Pg_Out : Outport  Port=2
  Pitch_Out : Outport  Port=3
  wires:
  MATLAB Function1/1(y) -> Manual Switch1/2
  MATLAB Function2/1(y) -> Mux/3, Mux/1, Mux/2
  Omega_g/1 -> Divide1/2
  MATLAB Function5/1(y) -> Pg_Out/1, Divide1/1
  Tg_In/1 -> MATLAB Function1/1(u)
  Divide1/1 -> Manual Switch1/1
  Clock2/1 -> MATLAB Function2/2(t)
  Clock5/1 -> MATLAB Function5/2(t)
  Pg_In/1 -> MATLAB Function5/1(u)
  Clock1/1 -> MATLAB Function1/2(t)
  Manual Switch1/1 -> Tg_Out/1
  Pitch_In/1 -> MATLAB Function2/1(u)
  Mux/1 -> Pitch_Out/1

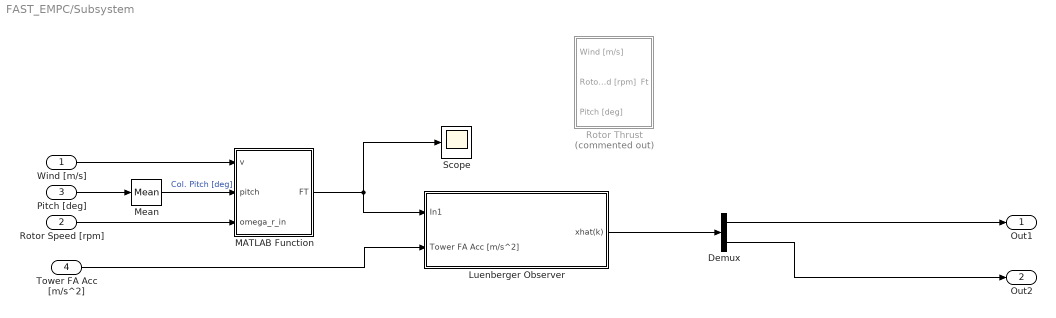
== system FAST_EMPC/Subsystem ==
  Wind [m/s] : Inport
  Rotor Speed [rpm] : Inport  Port=2
  Pitch [deg] : Inport  Port=3
  Tower FA Acc [m/s^2] : Inport  Port=4
  Demux : Demux  Outputs=2
  Luenberger Observer : Subsystem
  MATLAB Function : MATLAB Function  TreatAsAtomicUnit=on
  Mean : dspstat3/Mean  run=off  InputProcessing=Columns as channels (frame based)  reset_popup=None  directionMode=Entire input  dimension=1  roiEnable=off  roiType=Rectangles  roiPortion=Entire ROI  roiOutput=Individual statistics for each ROI  roiFlag=off  roundingMode=Floor  overflowMode=off  outputDataTypeStr=Inherit: Same as accumulator  outputMin=[]  outputMax=[]  outputLastDataTypeStr=Inherit: Same as accumulator
  Rotor Thrust : Subsystem  Commented=on
  Scope : Scope
  Out1 : Outport
  Out2 : Outport  Port=2
  wires:
  Luenberger Observer/1(xhat(k)) -> Demux/1
  Tower FA Acc [m/s^2]/1 -> Luenberger Observer/2(Tower FA Acc [m/s^2])
  MATLAB Function/1(FT) -> Scope/1, Luenberger Observer/1(In1)
  Demux/1 -> Out1/1
  Wind [m/s]/1 -> MATLAB Function/1(v)
  Demux/2 -> Out2/1
  Rotor Speed [rpm]/1 -> MATLAB Function/3(omega_r_in)
  Pitch [deg]/1 -> Mean/1
  Mean/1 -> MATLAB Function/2(pitch)  "Col. Pitch [deg]"

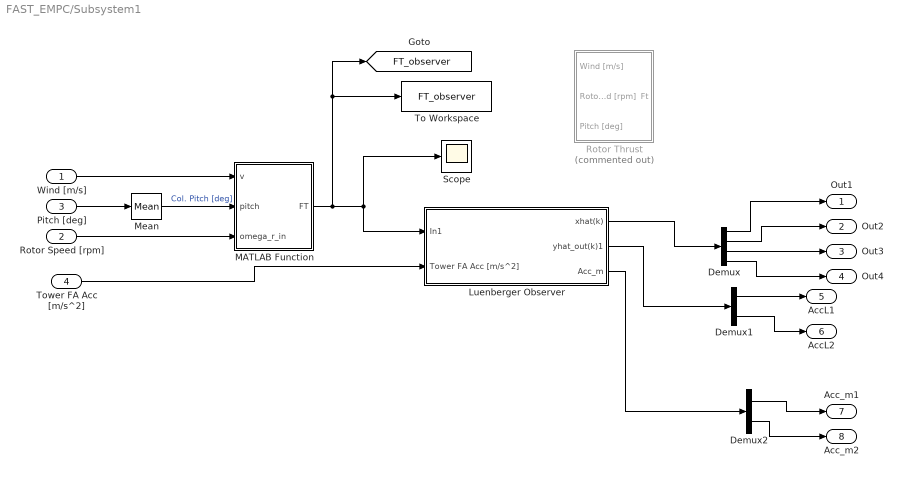
== system FAST_EMPC/Subsystem1 ==
  Wind [m/s] : Inport
  Rotor Speed [rpm] : Inport  Port=2
  Pitch [deg] : Inport  Port=3
  Tower FA Acc [m/s^2] : Inport  Port=4
  Demux : Demux
  Demux1 : Demux  Outputs=2
  Demux2 : Demux  Outputs=2
  Luenberger Observer : Subsystem
  MATLAB Function : MATLAB Function  TreatAsAtomicUnit=on
  Mean : dspstat3/Mean  run=off  InputProcessing=Columns as channels (frame based)  reset_popup=None  directionMode=Entire input  dimension=1  roiEnable=off  roiType=Rectangles  roiPortion=Entire ROI  roiOutput=Individual statistics for each ROI  roiFlag=off  roundingMode=Floor  overflowMode=off  outputDataTypeStr=Inherit: Same as accumulator  outputMin=[]  outputMax=[]  outputLastDataTypeStr=Inherit: Same as accumulator
  Rotor Thrust : Subsystem  Commented=on
  Scope : Scope
  To Workspace : ToWorkspace  VariableName=FT_observer  SaveFormat=Timeseries  SampleTime=-1
  Out1 : Outport
  Out2 : Outport  Port=2
  Out3 : Outport  Port=3
  Out4 : Outport  Port=4
  AccL1 : Outport  Port=5
  AccL2 : Outport  Port=6
  Acc_m1 : Outport  Port=7
  Acc_m2 : Outport  Port=8
  tag scope: FT_observer=global
  wires:
  Luenberger Observer/1(xhat(k)) -> Demux/1
  Tower FA Acc [m/s^2]/1 -> Luenberger Observer/2(Tower FA Acc [m/s^2])
  MATLAB Function/1(FT) -> [FT_observer], To Workspace/1, Scope/1, Luenberger Observer/1(In1)
  Demux/1 -> Out1/1
  Wind [m/s]/1 -> MATLAB Function/1(v)
  Demux/2 -> Out2/1
  Rotor Speed [rpm]/1 -> MATLAB Function/3(omega_r_in)
  Pitch [deg]/1 -> Mean/1
  Mean/1 -> MATLAB Function/2(pitch)  "Col. Pitch [deg]"
  Demux/3 -> Out3/1
  Demux/4 -> Out4/1
  Luenberger Observer/2(yhat_out(k)1) -> Demux1/1
  Demux1/1 -> AccL1/1
  Demux1/2 -> AccL2/1
  Demux2/2 -> Acc_m2/1
  Demux2/1 -> Acc_m1/1
  Luenberger Observer/3(Acc_m) -> Demux2/1

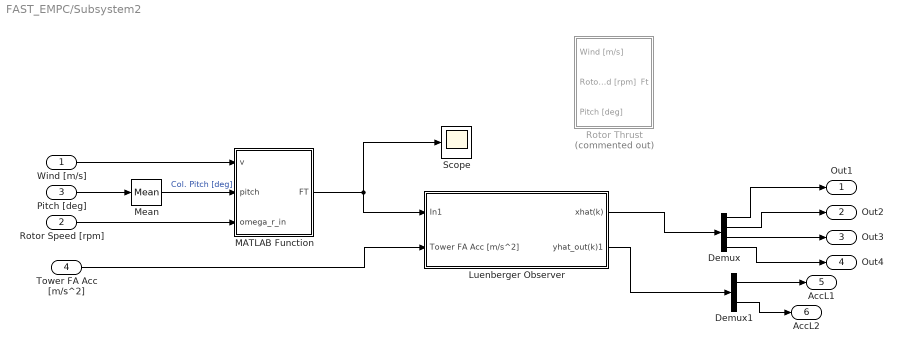
== system FAST_EMPC/Subsystem2 ==
  Wind [m/s] : Inport
  Rotor Speed [rpm] : Inport  Port=2
  Pitch [deg] : Inport  Port=3
  Tower FA Acc [m/s^2] : Inport  Port=4
  Demux : Demux
  Demux1 : Demux  Outputs=2
  Luenberger Observer : Subsystem
  MATLAB Function : MATLAB Function  TreatAsAtomicUnit=on
  Mean : dspstat3/Mean  run=off  InputProcessing=Columns as channels (frame based)  reset_popup=None  directionMode=Entire input  dimension=1  roiEnable=off  roiType=Rectangles  roiPortion=Entire ROI  roiOutput=Individual statistics for each ROI  roiFlag=off  roundingMode=Floor  overflowMode=off  outputDataTypeStr=Inherit: Same as accumulator  outputMin=[]  outputMax=[]  outputLastDataTypeStr=Inherit: Same as accumulator
  Rotor Thrust : Subsystem  Commented=on
  Scope : Scope
  Out1 : Outport
  Out2 : Outport  Port=2
  Out3 : Outport  Port=3
  Out4 : Outport  Port=4
  AccL1 : Outport  Port=5
  AccL2 : Outport  Port=6
  wires:
  Luenberger Observer/1(xhat(k)) -> Demux/1
  Tower FA Acc [m/s^2]/1 -> Luenberger Observer/2(Tower FA Acc [m/s^2])
  MATLAB Function/1(FT) -> Scope/1, Luenberger Observer/1(In1)
  Demux/1 -> Out1/1
  Wind [m/s]/1 -> MATLAB Function/1(v)
  Demux/2 -> Out2/1
  Rotor Speed [rpm]/1 -> MATLAB Function/3(omega_r_in)
  Pitch [deg]/1 -> Mean/1
  Mean/1 -> MATLAB Function/2(pitch)  "Col. Pitch [deg]"
  Demux/3 -> Out3/1
  Demux/4 -> Out4/1
  Luenberger Observer/2(yhat_out(k)1) -> Demux1/1
  Demux1/1 -> AccL1/1
  Demux1/2 -> AccL2/1

== system FAST_EMPC/Yaw and Yaw rate ==
  Mux : Mux  Inputs=2
  yaw : Constant  Value=0
  yaw rate : Constant  Value=0
  Out1 : Outport
  wires:
  yaw rate/1 -> Mux/2
  Mux/1 -> Out1/1
  yaw/1 -> Mux/1

== system FAST_EMPC/EMPC/Pav Coefficients ==
  vi : Inport
  Constraints_PW1 : MATLAB Function  TreatAsAtomicUnit=on  SystemSampleTime=Parameters.TsMPC
  IC : InitialCondition  Value=8
  Rate Transition : RateTransition
  first col of vi : MATLABFcn  MATLABFcn=u(1)  OutputDimensions=1
  AA : Outport
  BB : Outport  Port=2
  vi(1) : Outport  Port=3
  wires:
  vi/1 -> first col of vi/1
  Constraints_PW1/1(AA) -> AA/1
  Constraints_PW1/2(BB) -> BB/1
  first col of vi/1 -> IC/1, vi(1)/1
  IC/1 -> Rate Transition/1
  Rate Transition/1 -> Constraints_PW1/1(currentV)

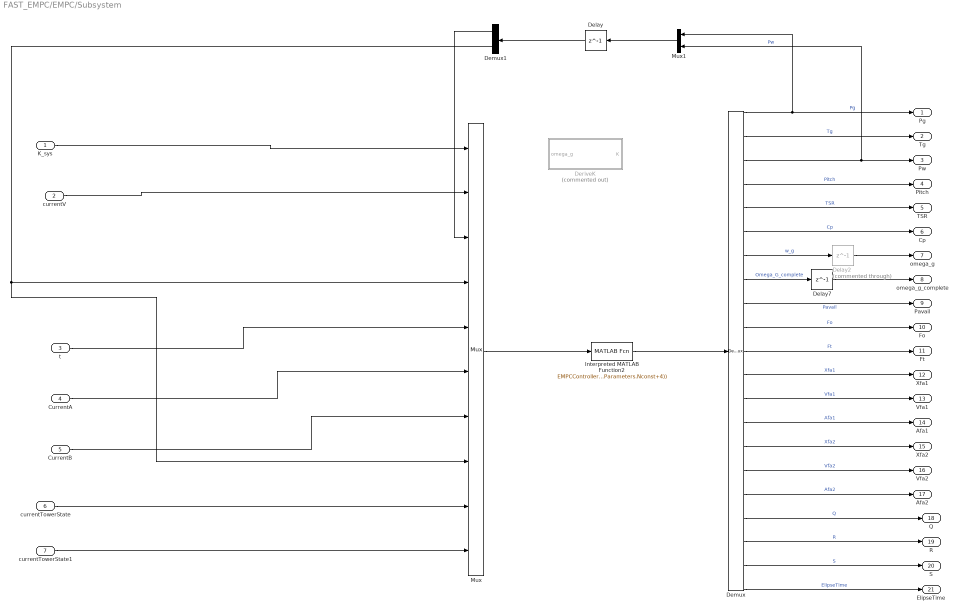
== system FAST_EMPC/EMPC/Subsystem ==
  K_sys : Inport
  currentV : Inport  Port=2
  t : Inport  Port=3
  CurrentA : Inport  Port=4
  CurrentB : Inport  Port=5
  currentTowerState : Inport  Port=6
  currentTowerState1 : Inport  Port=7
  Delay : Delay  DelayLength=1  InitialCondition=0
  Delay2 : Delay  Commented=through  DelayLength=1  InitialCondition=41.647046611088690  SampleTime=Parameters.Ts
  Delay7 : Delay  DelayLength=1  InitialCondition=1878726.43646583  SampleTime=0.2
  Demux : Demux  Outputs=[1 1 1 1 1 1 1 100 1 1 1 1 1 1 1 1 1 1 1 1 -1]
      settings: DisplayOption=none
  Demux1 : Demux  Outputs=2
  DeriveK : MATLAB Function  Commented=on  TreatAsAtomicUnit=on  SystemSampleTime=Parameters.DT
  Interpreted MATLAB Function2 : MATLABFcn  MATLABFcn=EMPCController_Tower(u(1),u(2),u(3),u(4),u(5),u(6:1:6+Parameters.Nconst-1),u(6+Parameters.Nconst:1:6+2*Parameters.Nconst-1),u(6+2*Parameters.Nconst),u(6+2*Parameters.Nconst+1:6+2*Parameters.Nconst+2),u(6+2*Parameters.Nconst+3:6+2*Parameters.Nconst+4))
  Mux : Mux  Inputs=10
  Mux1 : Mux  Inputs=2
  Pg : Outport
  Tg : Outport  Port=2
  Pw : Outport  Port=3
  Pitch : Outport  Port=4
  TSR : Outport  Port=5
  Cp : Outport  Port=6
  omega_g : Outport  Port=7
  omega_g_complete : Outport  Port=8
  Pavail : Outport  Port=9
  Fo : Outport  Port=10
  Ft : Outport  Port=11
  Xfa1 : Outport  Port=12
  Vfa1 : Outport  Port=13
  Afa1 : Outport  Port=14
  Xfa2 : Outport  Port=15
  Vfa2 : Outport  Port=16
  Afa2 : Outport  Port=17
  Q : Outport  Port=18
  R : Outport  Port=19
  S : Outport  Port=20
  ElipseTime : Outport  Port=21
  wires:
  Mux/1 -> Interpreted MATLAB Function2/1
  Demux1/2 -> Mux/8, Mux/4
  Demux1/1 -> Mux/3
  currentTowerState/1 -> Mux/9
  CurrentB/1 -> Mux/7
  t/1 -> Mux/5
  K_sys/1 -> Mux/1
  currentV/1 -> Mux/2
  CurrentA/1 -> Mux/6
  Mux1/1 -> Delay/1
  Delay/1 -> Demux1/1
  currentTowerState1/1 -> Mux/10
  Delay2/1 -> omega_g/1
  Demux/11 -> Ft/1  "Ft"
  Demux/1 -> Mux1/1, Pg/1  "Pg"
  Demux/8 -> Delay7/1  "Omega_G_complete"
  Demux/9 -> Pavail/1  "Pavail"
  Demux/15 -> Xfa2/1  "Xfa2"
  Demux/19 -> R/1  "R"
  Demux/4 -> Pitch/1  "Pitch"
  Demux/2 -> Tg/1  "Tg"
  Demux/7 -> Delay2/1  "w_g"
  Demux/21 -> ElipseTime/1  "ElipseTime"
  Demux/18 -> Q/1  "Q"
  Demux/12 -> Xfa1/1  "Xfa1"
  Demux/3 -> Mux1/2, Pw/1  "Pw"
  Demux/6 -> Cp/1  "Cp"
  Demux/5 -> TSR/1  "TSR"
  Demux/13 -> Vfa1/1  "Vfa1"
  Demux/20 -> S/1  "S"
  Demux/14 -> Afa1/1  "Afa1"
  Demux/17 -> Afa2/1  "Afa2"
  Demux/10 -> Fo/1  "Fo"
  Delay7/1 -> omega_g_complete/1
  Demux/16 -> Vfa2/1  "Vfa2"
  Interpreted MATLAB Function2/1 -> Demux/1

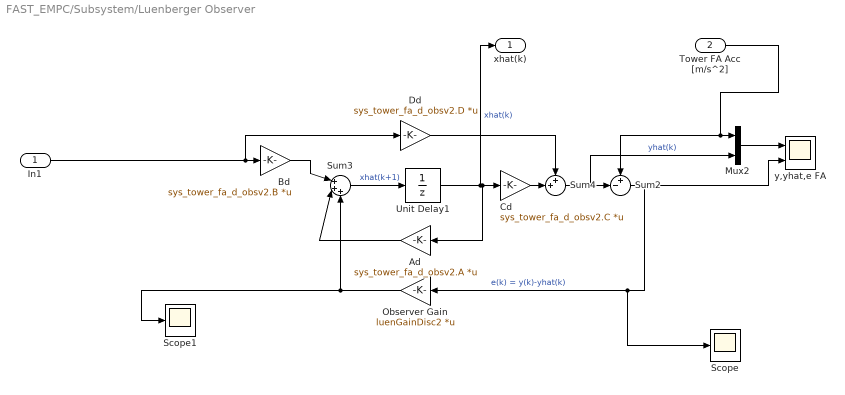
== system FAST_EMPC/Subsystem/Luenberger Observer ==
  In1 : Inport
  Tower FA Acc [m/s^2] : Inport  Port=2
  Ad : Gain  Gain=sys_tower_fa_d_obsv2.A  Multiplication=Matrix(K*u)
  Bd : Gain  Gain=sys_tower_fa_d_obsv2.B  Multiplication=Matrix(K*u)
  Cd : Gain  Gain=sys_tower_fa_d_obsv2.C  Multiplication=Matrix(K*u)
  Dd : Gain  Gain=sys_tower_fa_d_obsv2.D  Multiplication=Matrix(K*u)
  Mux2 : Mux  Inputs=2
  Observer Gain : Gain  Gain=luenGainDisc2  Multiplication=Matrix(K*u)
  Scope : Scope
  Scope1 : Scope
  Sum2 : Sum  Inputs=+-|
  Sum3 : Sum  Inputs=|+++
  Sum4 : Sum  Inputs=++|
  Unit Delay1 : UnitDelay  SampleTime=-1  HasFrameUpgradeWarning=on
  y,yhat,e FA : Scope  NumInputPorts=2
  xhat(k) : Outport
  wires:
  Sum3/1 -> Unit Delay1/1  "xhat(k+1)"
  Unit Delay1/1 -> xhat(k)/1, Ad/1, Cd/1  "xhat(k)"
  Observer Gain/1 -> Sum3/3, Scope1/1
  Sum4/1 -> Sum2/2, Mux2/2  "yhat(k)"
  Tower FA Acc [m/s^2]/1 -> Sum2/1, Mux2/1
  Cd/1 -> Sum4/2
  Sum2/1 -> Observer Gain/1, Scope/1, y,yhat,e FA/2  "e(k) = y(k)-yhat(k)"
  In1/1 -> Bd/1, Dd/1
  Dd/1 -> Sum4/1
  Ad/1 -> Sum3/2
  Mux2/1 -> y,yhat,e FA/1
  Bd/1 -> Sum3/1

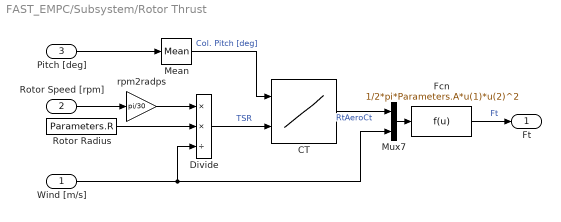
== system FAST_EMPC/Subsystem/Rotor Thrust ==
  Wind [m/s] : Inport
  Rotor Speed [rpm] : Inport  Port=2
  Pitch [deg] : Inport  Port=3
  CT : Lookup_n-D  BreakpointsForDimension1=Parameters.Rotor_PitchFull  BreakpointsForDimension2=Parameters.Rotor_Lamda  Table=Parameters.Rotor_cTFull  InternalRulePriority=Speed  RndMeth=Simplest  InputSameDT=on
      settings: InputPortMap=u0,u1
  Divide : Product  Inputs=**/
  Fcn : Fcn  Expr=1/2*pi*Parameters.A*u(1)*u(2)^2
  Mean : dspstat3/Mean  run=off  InputProcessing=Columns as channels (frame based)  reset_popup=None  directionMode=Entire input  dimension=1  roiEnable=off  roiType=Rectangles  roiPortion=Entire ROI  roiOutput=Individual statistics for each ROI  roiFlag=off  roundingMode=Floor  overflowMode=off  outputDataTypeStr=Inherit: Same as accumulator  outputMin=[]  outputMax=[]  outputLastDataTypeStr=Inherit: Same as accumulator
  Mux7 : Mux  Inputs=2
  Rotor Radius : Constant  Value=Parameters.R
  rpm2radps : Gain  Gain=pi/30
  Ft : Outport
  wires:
  Fcn/1 -> Ft/1  "Ft"
  Mean/1 -> CT/1  "Col. Pitch [deg]"
  Mux7/1 -> Fcn/1
  CT/1 -> Mux7/1  "RtAeroCt"
  Pitch [deg]/1 -> Mean/1
  Wind [m/s]/1 -> Divide/3, Mux7/2
  Divide/1 -> CT/2  "TSR"
  rpm2radps/1 -> Divide/1
  Rotor Radius/1 -> Divide/2
  Rotor Speed [rpm]/1 -> rpm2radps/1

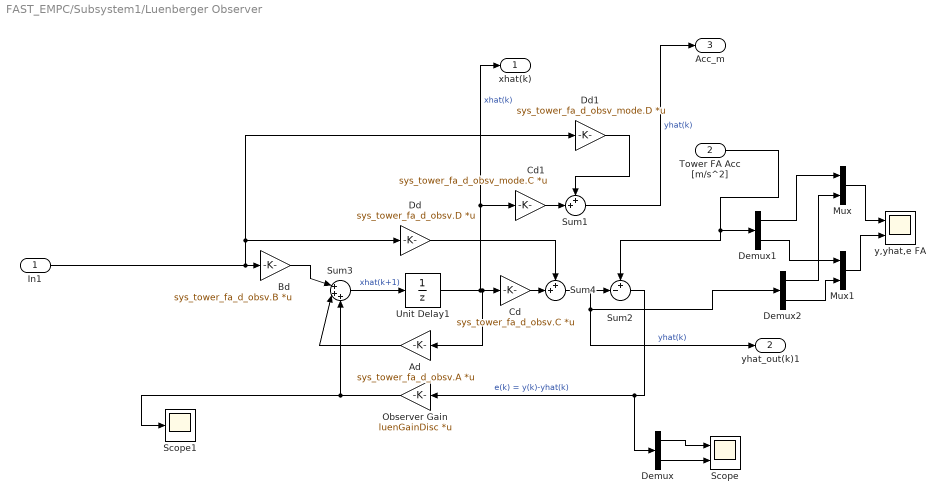
== system FAST_EMPC/Subsystem1/Luenberger Observer ==
  In1 : Inport
  Tower FA Acc [m/s^2] : Inport  Port=2
  Ad : Gain  Gain=sys_tower_fa_d_obsv.A  Multiplication=Matrix(K*u)
  Bd : Gain  Gain=sys_tower_fa_d_obsv.B  Multiplication=Matrix(K*u)
  Cd : Gain  Gain=sys_tower_fa_d_obsv.C  Multiplication=Matrix(K*u)
  Cd1 : Gain  Gain=sys_tower_fa_d_obsv_mode.C  Multiplication=Matrix(K*u)
  Dd : Gain  Gain=sys_tower_fa_d_obsv.D  Multiplication=Matrix(K*u)
  Dd1 : Gain  Gain=sys_tower_fa_d_obsv_mode.D  Multiplication=Matrix(K*u)
  Demux : Demux  Outputs=2
  Demux1 : Demux  Outputs=2
  Demux2 : Demux  Outputs=2
  Mux : Mux  Inputs=2
  Mux1 : Mux  Inputs=2
  Observer Gain : Gain  Gain=luenGainDisc  Multiplication=Matrix(K*u)
  Scope : Scope  NumInputPorts=2
  Scope1 : Scope
  Sum1 : Sum  Inputs=++|
  Sum2 : Sum  Inputs=+-|
  Sum3 : Sum  Inputs=|+++
  Sum4 : Sum  Inputs=++|
  Unit Delay1 : UnitDelay  SampleTime=-1  HasFrameUpgradeWarning=on
  y,yhat,e FA : Scope  NumInputPorts=2
  xhat(k) : Outport
  yhat_out(k)1 : Outport  Port=2
  Acc_m : Outport  Port=3
  wires:
  Sum3/1 -> Unit Delay1/1  "xhat(k+1)"
  Unit Delay1/1 -> Cd1/1, xhat(k)/1, Ad/1, Cd/1  "xhat(k)"
  Observer Gain/1 -> Sum3/3, Scope1/1
  Sum4/1 -> Demux2/1, yhat_out(k)1/1, Sum2/2  "yhat(k)"
  Tower FA Acc [m/s^2]/1 -> Sum2/1, Demux1/1
  Cd/1 -> Sum4/2
  Sum2/1 -> Demux/1, Observer Gain/1  "e(k) = y(k)-yhat(k)"
  In1/1 -> Bd/1, Dd1/1, Dd/1
  Dd/1 -> Sum4/1
  Ad/1 -> Sum3/2
  Bd/1 -> Sum3/1
  Cd1/1 -> Sum1/2
  Dd1/1 -> Sum1/1
  Sum1/1 -> Acc_m/1  "yhat(k)"
  Demux/1 -> Scope/1
  Demux/2 -> Scope/2
  Demux1/1 -> Mux/1
  Demux2/1 -> Mux/2
  Demux1/2 -> Mux1/1
  Demux2/2 -> Mux1/2
  Mux1/1 -> y,yhat,e FA/2
  Mux/1 -> y,yhat,e FA/1

== system FAST_EMPC/Subsystem1/Rotor Thrust ==
  Wind [m/s] : Inport
  Rotor Speed [rpm] : Inport  Port=2
  Pitch [deg] : Inport  Port=3
  CT : Lookup_n-D  BreakpointsForDimension1=Parameters.Rotor_PitchFull  BreakpointsForDimension2=Parameters.Rotor_Lamda  Table=Parameters.Rotor_cTFull  InternalRulePriority=Speed  RndMeth=Simplest  InputSameDT=on
      settings: InputPortMap=u0,u1
  Divide : Product  Inputs=**/
  Fcn : Fcn  Expr=1/2*pi*Parameters.A*u(1)*u(2)^2
  Mean : dspstat3/Mean  run=off  InputProcessing=Columns as channels (frame based)  reset_popup=None  directionMode=Entire input  dimension=1  roiEnable=off  roiType=Rectangles  roiPortion=Entire ROI  roiOutput=Individual statistics for each ROI  roiFlag=off  roundingMode=Floor  overflowMode=off  outputDataTypeStr=Inherit: Same as accumulator  outputMin=[]  outputMax=[]  outputLastDataTypeStr=Inherit: Same as accumulator
  Mux7 : Mux  Inputs=2
  Rotor Radius : Constant  Value=Parameters.R
  rpm2radps : Gain  Gain=pi/30
  Ft : Outport
  wires:
  Fcn/1 -> Ft/1  "Ft"
  Mean/1 -> CT/1  "Col. Pitch [deg]"
  Mux7/1 -> Fcn/1
  CT/1 -> Mux7/1  "RtAeroCt"
  Pitch [deg]/1 -> Mean/1
  Wind [m/s]/1 -> Divide/3, Mux7/2
  Divide/1 -> CT/2  "TSR"
  rpm2radps/1 -> Divide/1
  Rotor Radius/1 -> Divide/2
  Rotor Speed [rpm]/1 -> rpm2radps/1

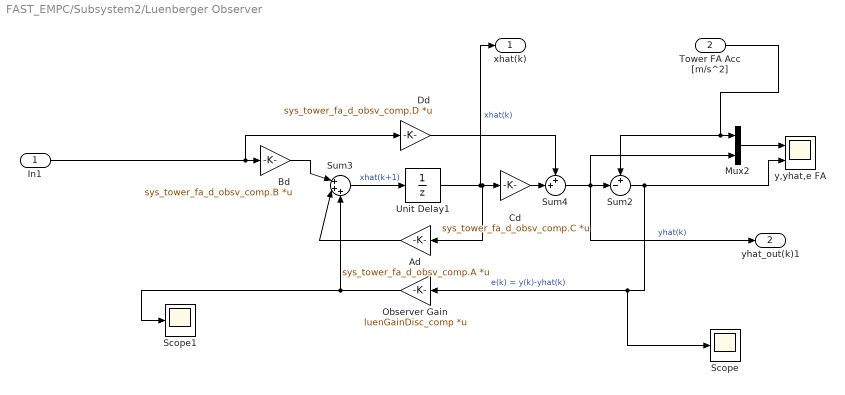
== system FAST_EMPC/Subsystem2/Luenberger Observer ==
  In1 : Inport
  Tower FA Acc [m/s^2] : Inport  Port=2
  Ad : Gain  Gain=sys_tower_fa_d_obsv_comp.A  Multiplication=Matrix(K*u)
  Bd : Gain  Gain=sys_tower_fa_d_obsv_comp.B  Multiplication=Matrix(K*u)
  Cd : Gain  Gain=sys_tower_fa_d_obsv_comp.C  Multiplication=Matrix(K*u)
  Dd : Gain  Gain=sys_tower_fa_d_obsv_comp.D  Multiplication=Matrix(K*u)
  Mux2 : Mux  Inputs=2
  Observer Gain : Gain  Gain=luenGainDisc_comp  Multiplication=Matrix(K*u)
  Scope : Scope
  Scope1 : Scope
  Sum2 : Sum  Inputs=+-|
  Sum3 : Sum  Inputs=|+++
  Sum4 : Sum  Inputs=++|
  Unit Delay1 : UnitDelay  SampleTime=-1  HasFrameUpgradeWarning=on
  y,yhat,e FA : Scope  NumInputPorts=2
  xhat(k) : Outport
  yhat_out(k)1 : Outport  Port=2
  wires:
  Sum3/1 -> Unit Delay1/1  "xhat(k+1)"
  Unit Delay1/1 -> xhat(k)/1, Ad/1, Cd/1  "xhat(k)"
  Observer Gain/1 -> Sum3/3, Scope1/1
  Sum4/1 -> yhat_out(k)1/1, Sum2/2, Mux2/2  "yhat(k)"
  Tower FA Acc [m/s^2]/1 -> Sum2/1, Mux2/1
  Cd/1 -> Sum4/2
  Sum2/1 -> Observer Gain/1, Scope/1, y,yhat,e FA/2  "e(k) = y(k)-yhat(k)"
  In1/1 -> Bd/1, Dd/1
  Dd/1 -> Sum4/1
  Ad/1 -> Sum3/2
  Mux2/1 -> y,yhat,e FA/1
  Bd/1 -> Sum3/1

== system FAST_EMPC/Subsystem2/Rotor Thrust ==
  Wind [m/s] : Inport
  Rotor Speed [rpm] : Inport  Port=2
  Pitch [deg] : Inport  Port=3
  CT : Lookup_n-D  BreakpointsForDimension1=Parameters.Rotor_PitchFull  BreakpointsForDimension2=Parameters.Rotor_Lamda  Table=Parameters.Rotor_cTFull  InternalRulePriority=Speed  RndMeth=Simplest  InputSameDT=on
      settings: InputPortMap=u0,u1
  Divide : Product  Inputs=**/
  Fcn : Fcn  Expr=1/2*pi*Parameters.A*u(1)*u(2)^2
  Mean : dspstat3/Mean  run=off  InputProcessing=Columns as channels (frame based)  reset_popup=None  directionMode=Entire input  dimension=1  roiEnable=off  roiType=Rectangles  roiPortion=Entire ROI  roiOutput=Individual statistics for each ROI  roiFlag=off  roundingMode=Floor  overflowMode=off  outputDataTypeStr=Inherit: Same as accumulator  outputMin=[]  outputMax=[]  outputLastDataTypeStr=Inherit: Same as accumulator
  Mux7 : Mux  Inputs=2
  Rotor Radius : Constant  Value=Parameters.R
  rpm2radps : Gain  Gain=pi/30
  Ft : Outport
  wires:
  Fcn/1 -> Ft/1  "Ft"
  Mean/1 -> CT/1  "Col. Pitch [deg]"
  Mux7/1 -> Fcn/1
  CT/1 -> Mux7/1  "RtAeroCt"
  Pitch [deg]/1 -> Mean/1
  Wind [m/s]/1 -> Divide/3, Mux7/2
  Divide/1 -> CT/2  "TSR"
  rpm2radps/1 -> Divide/1
  Rotor Radius/1 -> Divide/2
  Rotor Speed [rpm]/1 -> rpm2radps/1
